simulink library "TYPEBP_MASTER_tmp"  (Simulink 8.6)
settings: Solver=ode45  StartTime=0.0  StopTime=10.0  RelTol=1e-3
undefined symbols (not defined in the file): TYPEC, TYPEC_MASTER
libraries: cdsEpicsOut x112, cdsFilt x79, cdsTP x59, cdsFiltCtrl x36, VIS_LIB x20, cdsEpicsIn x18, cdsMuxMatrix x14, STATE_BIO_MASTER x12, cdsEpicsBinIn x8, cdsFunctionCall x4, lockin x4, cdsEpicsStringIn x2
(part 1 of 13)
settings Model: Creator=controls  LastModifiedBy=controls

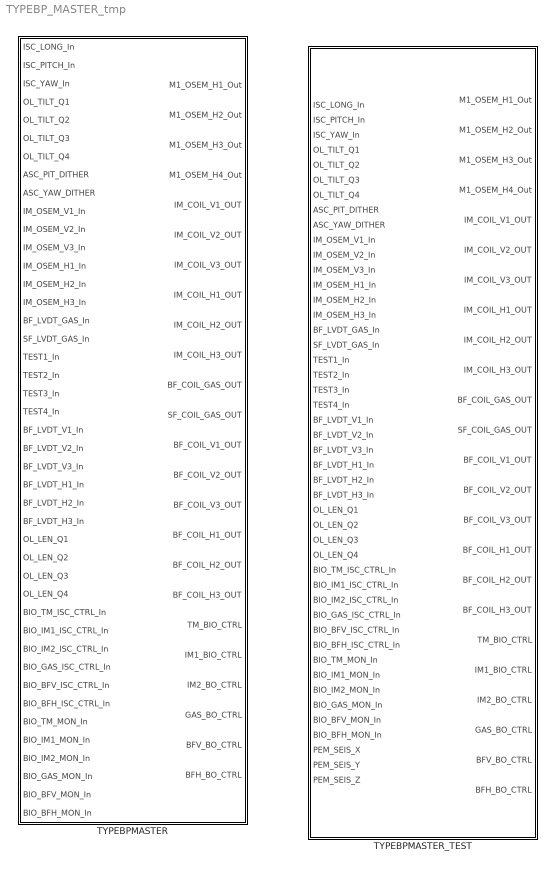
== system TYPEBP_MASTER_tmp ==
  TYPEBPMASTER : Subsystem  Description=TYPEBP MASTER  AncestorBlock=TYPEC_MASTER/TYPEC
      settings: AttributesFormatString=%<Description>
  TYPEBPMASTER_TEST : Subsystem  Description=TYPEBP MASTER
      settings: AttributesFormatString=%<Description>

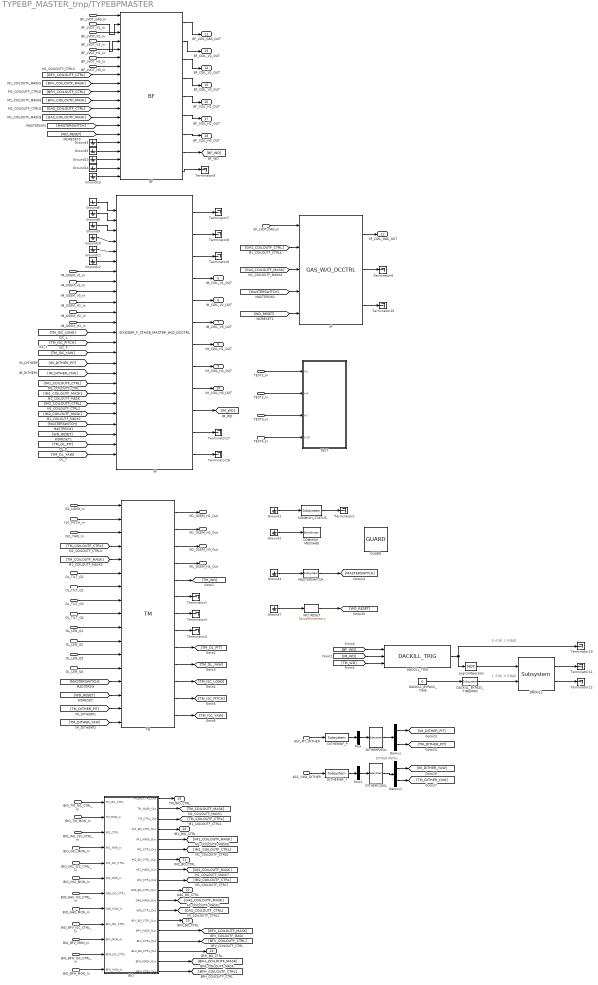
== system TYPEBP_MASTER_tmp/TYPEBPMASTER ==
  note: DITHER PATHs
      |
      |
      |
      |
      |
      |
      |
      |
      |
      |
      |
      |
      |
      |
      | .                                                                                                      .
  note: 0 if OK, 1 if BAD
  note: 1 if OK, 0 if BAD
  ISC_LONG_In : Inport
  ISC_PITCH_In : Inport  Port=2
  ISC_YAW_In : Inport  Port=3
  OL_TILT_Q1 : Inport  Port=4
  OL_TILT_Q2 : Inport  Port=5
  OL_TILT_Q3 : Inport  Port=6
  OL_TILT_Q4 : Inport  Port=7
  ASC_PIT_DITHER : Inport  Port=8
  ASC_YAW_DITHER : Inport  Port=9
  IM_OSEM_V1_In : Inport  Port=10
  IM_OSEM_V2_In : Inport  Port=11
  IM_OSEM_V3_In : Inport  Port=12
  IM_OSEM_H1_In : Inport  Port=13
  IM_OSEM_H2_In : Inport  Port=14
  IM_OSEM_H3_In : Inport  Port=15
  BF_LVDT_GAS_In : Inport  Port=16
  SF_LVDT_GAS_In : Inport  Port=17
  TEST1_In : Inport  Port=18
  TEST2_In : Inport  Port=19
  TEST3_In : Inport  Port=20
  TEST4_In : Inport  Port=21
  BF_LVDT_V1_In : Inport  Port=22
  BF_LVDT_V2_In : Inport  Port=23
  BF_LVDT_V3_In : Inport  Port=24
  BF_LVDT_H1_In : Inport  Port=25
  BF_LVDT_H2_In : Inport  Port=26
  BF_LVDT_H3_In : Inport  Port=27
  OL_LEN_Q1 : Inport  Port=28
  OL_LEN_Q2 : Inport  Port=29
  OL_LEN_Q3 : Inport  Port=30
  OL_LEN_Q4 : Inport  Port=31
  BIO_TM_ISC_CTRL_In : Inport  Port=32
  BIO_IM1_ISC_CTRL_In : Inport  Port=33
  BIO_IM2_ISC_CTRL_In : Inport  Port=34
  BIO_GAS_ISC_CTRL_In : Inport  Port=35
  BIO_BFV_ISC_CTRL_In : Inport  Port=36
  BIO_BFH_ISC_CTRL_In : Inport  Port=37
  BIO_TM_MON_In : Inport  Port=38
  BIO_IM1_MON_In : Inport  Port=39
  BIO_IM2_MON_In : Inport  Port=40
  BIO_GAS_MON_In : Inport  Port=41
  BIO_BFV_MON_In : Inport  Port=42
  BIO_BFH_MON_In : Inport  Port=43
  BF : BF_MASTER/BF
  BIO : Subsystem
  COMMISH_MESSAGE : cdsEpicsStringIn/EpicsStringIn  Tag=cdsEpicsStringIn  Description=cdsEpicsStringIn
      settings: AttributesFormatString=%<Tag>
  COMMISH_STATUS : cdsEpicsBinIn/Subsystem  Tag=cdsEpicsBinIn  Description=|
      | Purpose:                                                                            
      | Create an EPICS binary (0 or 1) input channel to the FE realtime controls.          
      |                                                                                     
      | Operation:                                                                          
      | Outputs value from an EPICS ai record. Value is binary input (bi Epics record type).
      |                                                                                     
      | Usage:                                                                              
      | Name the part with the desired EPICS channel name.
      settings: AttributesFormatString=%<Tag>
  DACKILL : cdsDacKill/Subsystem  Description=cdsDacKill
      settings: AttributesFormatString=%<Description>
  DACKILL_BYPASS_TIME : Constant  Value=0
  DACKILL_BYPASS_TIMEMON : cdsEpicsOut/Subsystem  Tag=cdsEpicsOutput  Description=|
      | Purpose:                                          
      | Output a FE signal to an EPICS channel.           
      |                                                   
      | Operation:                                        
      | Takes input value and passes it to EPICS record.  
      |                                                   
      | Usage:                                            
      | Name the part with the desired EPICS rrecord name.
      settings: AttributesFormatString=%<Tag>
  DACKILL_TRIG : VIS_LIB/DACKILL_TRIG
  DITHERINF_P : cdsFilt/Subsystem  Tag=cdsFilt  Description=|
      | Purpose:                                                                                                                                                                                                                                  
      | Standard CDS IIR filter module.                                                                                                                                                                                                           
      |                                                                                                                                                                                                                                           
      | Operation:                                                                                                                                                                                                                                
      | Consists of 10 second order section IIR filters, plus a ramped gain stage. In FE code, also provides pre-defined test points and excitation channel inputs. The filter coefficients are defined in the LIGO system using the 'foton' tool.
      |                                                                                                                                                                                                                                           
      | Usage:                                                                                                                                                                                                                                    
      | Name the part with the desired filter module name.
      settings: AttributesFormatString=%<Tag>
  DITHERINF_Y : cdsFilt/Subsystem  Tag=cdsFilt  Description=|
      | Purpose:                                                                                                                                                                                                                                  
      | Standard CDS IIR filter module.                                                                                                                                                                                                           
      |                                                                                                                                                                                                                                           
      | Operation:                                                                                                                                                                                                                                
      | Consists of 10 second order section IIR filters, plus a ramped gain stage. In FE code, also provides pre-defined test points and excitation channel inputs. The filter coefficients are defined in the LIGO system using the 'foton' tool.
      |                                                                                                                                                                                                                                           
      | Usage:                                                                                                                                                                                                                                    
      | Name the part with the desired filter module name.
      settings: AttributesFormatString=%<Tag>
  DITHERP2EUL : cdsMuxMatrix/Subsystem  Tag=cdsMuxMatrix  Description=Any size matrix. Inputs and outputs must be connected using Mux and Demux parts.
      settings: AttributesFormatString=%<Tag>
  DITHERY2EUL : cdsMuxMatrix/Subsystem  Tag=cdsMuxMatrix  Description=Any size matrix. Inputs and outputs must be connected using Mux and Demux parts.
      settings: AttributesFormatString=%<Tag>
  Demux : Demux  Outputs=2
  Demux1 : Demux  Outputs=2
  GUARD : ISC_common/GUARD
  Ground{1..15} (15 alike) : Ground
  IM : SIXOSEM_F_STAGE_MASTER/SIXOSEM_F_STAGE_MASTER_W//O_DCCTRL  Description=SIXOSEMSTAGE_FACE_MASTER
  LogicalOperator : Logic  Operator=NOT  AllPortsSameDT=off  OutDataTypeStr=boolean
  MASTERSWITCH : cdsEpicsBinIn/Subsystem  Tag=cdsEpicsBinIn  Description=|
      | Purpose:                                                                            
      | Create an EPICS binary (0 or 1) input channel to the FE realtime controls.          
      |                                                                                     
      | Operation:                                                                          
      | Outputs value from an EPICS ai record. Value is binary input (bi Epics record type).
      |                                                                                     
      | Usage:                                                                              
      | Name the part with the desired EPICS channel name.
      settings: AttributesFormatString=%<Tag>
  Mux : Mux  Inputs=1
  Mux1 : Mux  Inputs=1
  SF : GAS_MASTER/GAS_W//O_DCCTRL
  TEST : Subsystem
  TM : TM_MASTER/TM
  Terminator{1..12,17..19} (15 alike) : Terminator
  WD_RESET : cdsEpicsMomentary/EpicsMomentary  Tag=cdsEpicsMomentary
      settings: AttributesFormatString=%<Tag>
  M1_OSEM_H1_Out : Outport
  M1_OSEM_H2_Out : Outport  Port=2
  M1_OSEM_H3_Out : Outport  Port=3
  M1_OSEM_H4_Out : Outport  Port=4
  IM_COIL_V1_OUT : Outport  Port=5
  IM_COIL_V2_OUT : Outport  Port=6
  IM_COIL_V3_OUT : Outport  Port=7
  IM_COIL_H1_OUT : Outport  Port=8
  IM_COIL_H2_OUT : Outport  Port=9
  IM_COIL_H3_OUT : Outport  Port=10
  BF_COIL_GAS_OUT : Outport  Port=11
  SF_COIL_GAS_OUT : Outport  Port=12
  BF_COIL_V1_OUT : Outport  Port=13
  BF_COIL_V2_OUT : Outport  Port=14
  BF_COIL_V3_OUT : Outport  Port=15
  BF_COIL_H1_OUT : Outport  Port=16
  BF_COIL_H2_OUT : Outport  Port=17
  BF_COIL_H3_OUT : Outport  Port=18
  TM_BIO_CTRL : Outport  Port=19
  IM1_BIO_CTRL : Outport  Port=20
  IM2_BO_CTRL : Outport  Port=21
  GAS_BO_CTRL : Outport  Port=22
  BFV_BO_CTRL : Outport  Port=23
  BFH_BO_CTRL : Outport  Port=24
  wires:
  [TM_COILOUTF_MASK] -> TM/5
  [TM_COILOUTF_CTRL] -> TM/4
  [WD_RESET] -> TM/15
  WD_RESET/1 -> [WD_RESET]
  Ground7/1 -> WD_RESET/1
  TM/6 -> Terminator1/1
  TM/7 -> Terminator3/1
  TM/8 -> Terminator4/1
  [MASTERSWITCH] -> TM/14
  OL_TILT_Q4/1 -> TM/9
  ISC_YAW_In/1 -> TM/3
  ISC_PITCH_In/1 -> TM/2
  OL_TILT_Q3/1 -> TM/8
  OL_TILT_Q2/1 -> TM/7
  OL_TILT_Q1/1 -> TM/6
  Ground4/1 -> MASTERSWITCH/1
  MASTERSWITCH/1 -> [MASTERSWITCH]
  TM/4 -> M1_OSEM_H4_Out/1
  TM/3 -> M1_OSEM_H3_Out/1
  TM/2 -> M1_OSEM_H2_Out/1
  TM/5 -> [TM_WD]
  ISC_LONG_In/1 -> TM/1
  Ground2/1 -> COMMISH_MESSAGE/1
  COMMISH_STATUS/1 -> Terminator2/1
  Ground1/1 -> COMMISH_STATUS/1
  ASC_YAW_DITHER/1 -> DITHERINF_Y/1
  Mux/1 -> DITHERP2EUL/1
  DITHERP2EUL/1 -> Demux/1
  ASC_PIT_DITHER/1 -> DITHERINF_P/1
  Mux1/1 -> DITHERY2EUL/1
  DITHERY2EUL/1 -> Demux1/1
  Demux/1 -> [IM_DITHER_PIT]
  Demux/2 -> [TM_DITHER_PIT]
  Demux1/1 -> [IM_DITHER_YAW]
  Demux1/2 -> [TM_DITHER_YAW]
  DITHERINF_P/1 -> Mux/1
  DITHERINF_Y/1 -> Mux1/1
  [TM_DITHER_PIT] -> TM/16
  [TM_DITHER_YAW] -> TM/17
  Ground9/1 -> IM/3
  Ground11/1 -> IM/5
  Ground6/1 -> IM/1
  Ground8/1 -> IM/2
  [TM_ISC_LONG] -> IM/13
  Ground10/1 -> IM/4
  Ground12/1 -> IM/6
  [TM_ISC_PITCH] -> IM/14
  [TM_ISC_YAW] -> IM/15
  IM/1 -> Terminator7/1
  IM/10 -> [IM_WD]
  IM/11 -> Terminator17/1
  IM/2 -> Terminator8/1
  IM/3 -> Terminator9/1
  IM/12 -> Terminator18/1
  IM_OSEM_V3_In/1 -> IM/9
  IM_OSEM_V2_In/1 -> IM/8
  IM_OSEM_V1_In/1 -> IM/7
  IM_OSEM_H3_In/1 -> IM/12
  IM_OSEM_H2_In/1 -> IM/11
  IM_OSEM_H1_In/1 -> IM/10
  IM/4 -> IM_COIL_V1_OUT/1
  IM/5 -> IM_COIL_V2_OUT/1
  IM/6 -> IM_COIL_V3_OUT/1
  IM/7 -> IM_COIL_H1_OUT/1
  IM/8 -> IM_COIL_H2_OUT/1
  IM/9 -> IM_COIL_H3_OUT/1
  TEST3_In/1 -> TEST/3(In7)
  TEST2_In/1 -> TEST/2(In4)
  TEST1_In/1 -> TEST/1(In1)
  TEST4_In/1 -> TEST/4(In10)
  TM/1 -> M1_OSEM_H1_Out/1
  [TM_WD] -> DACKILL_TRIG/3
  DACKILL_TRIG/1 -> Terminator19/1, LogicalOperator/1
  LogicalOperator/1 -> DACKILL/1
  DACKILL_BYPASS_TIMEMON/1 -> DACKILL/2
  DACKILL_BYPASS_TIME/1 -> DACKILL_BYPASS_TIMEMON/1
  DACKILL/1 -> Terminator11/1
  DACKILL/2 -> Terminator12/1
  [IM_WD] -> DACKILL_TRIG/2
  [IM1_COILOUTF_CTRL] -> IM/18
  [IM_DITHER_PIT] -> IM/16
  [IM_DITHER_YAW] -> IM/17
  [IM1_COILOUTF_MASK] -> IM/19
  TM/9 -> [TM_OL_PIT]
  TM/10 -> [TM_OL_YAW]
  [BF_WD] -> DACKILL_TRIG/1
  OL_LEN_Q4/1 -> TM/13
  OL_LEN_Q3/1 -> TM/12
  OL_LEN_Q2/1 -> TM/11
  OL_LEN_Q1/1 -> TM/10
  [BFV_COILOUTF_MASK] -> BF/9
  [BFV_COILOUTF_CTRL] -> BF/8
  BF_LVDT_H3_In/1 -> BF/7
  BF_LVDT_H2_In/1 -> BF/6
  BF_LVDT_H1_In/1 -> BF/5
  BF_LVDT_V3_In/1 -> BF/4
  BF_LVDT_V2_In/1 -> BF/3
  BF_LVDT_V1_In/1 -> BF/2
  BF_LVDT_GAS_In/1 -> BF/1
  BF/1 -> BF_COIL_GAS_OUT/1
  BF/2 -> BF_COIL_V1_OUT/1
  BF/3 -> BF_COIL_V2_OUT/1
  BF/4 -> BF_COIL_V3_OUT/1
  BF/5 -> BF_COIL_H1_OUT/1
  BF/6 -> BF_COIL_H2_OUT/1
  BF/7 -> BF_COIL_H3_OUT/1
  BF/9 -> Terminator5/1
  BF/8 -> [BF_WD]
  [GAS_COILOUTF_CTRL] -> SF/2
  [GAS_COILOUTF_MASK] -> SF/3
  [MASTERSWITCH] -> SF/4
  [WD_RESET] -> SF/5
  SF_LVDT_GAS_In/1 -> SF/1
  SF/2 -> Terminator6/1
  SF/1 -> SF_COIL_GAS_OUT/1
  SF/3 -> Terminator10/1
  BIO/12(GAS_CTRL_Out) -> [GAS_COILOUTF_CTRL]
  BIO/11(GAS_MASK_Out) -> [GAS_COILOUTF_MASK]
  BIO/3(TM_CTRL_Out) -> [TM_COILOUTF_CTRL]
  BIO/2(TM_MASK_Out) -> [TM_COILOUTF_MASK]
  BIO/6(IM1_CTRL_Out) -> [IM1_COILOUTF_CTRL]
  BIO/5(IM1_MASK_Out) -> [IM1_COILOUTF_MASK]
  BIO/13(BFV_BO_CTRL_Out) -> BFV_BO_CTRL/1
  BIO/10(GAS_BO_CTRL_Out) -> GAS_BO_CTRL/1
  BIO/7(IM2_BO_CTRL_Out) -> IM2_BO_CTRL/1
  BIO/4(IM1_BO_CTRL_Out) -> IM1_BIO_CTRL/1
  BIO/1(TM_BO_CTRL_Out) -> TM_BIO_CTRL/1
  BIO_GAS_MON_In/1 -> BIO/8(GAS_MON_In)
  BIO_GAS_ISC_CTRL_In/1 -> BIO/7(GAS_ISC_CTRL)
  BIO_IM2_MON_In/1 -> BIO/6(IM2_MON_In)
  BIO_IM2_ISC_CTRL_In/1 -> BIO/5(IM2_ISC_CTRL)
  BIO_IM1_MON_In/1 -> BIO/4(IM1_MON_In)
  BIO_IM1_ISC_CTRL_In/1 -> BIO/3(IM1_CTRL)
  BIO_TM_MON_In/1 -> BIO/2(TM_MON_In)
  BIO_TM_ISC_CTRL_In/1 -> BIO/1(TM_ISC_CTRL)
  BIO/8(IM2_MASK_Out) -> [IM2_COILOUTF_MASK]
  BIO/9(IM2_CTRL_Out) -> [IM2_COILOUTF_CTRL]
  BIO_BFV_ISC_CTRL_In/1 -> BIO/9(BFV_ISC_CTRL)
  BIO_BFV_MON_In/1 -> BIO/10(BFV_MON_In)
  BIO_BFH_ISC_CTRL_In/1 -> BIO/11(BFH_ISC_CTRL)
  BIO_BFH_MON_In/1 -> BIO/12(BFH_MON_In)
  BIO/14(BFV_MASK_Out) -> [BFV_COILOUTF_MASK]
  BIO/15(BFV_CTRL_Out) -> [BFV_COILOUTF_CTRL]
  BIO/17(BFH_MASK_Out) -> [BFH_COILOUTF_MASK]
  BIO/18(BFH_CTRL_Out) -> [BFH_COILOUTF_CTRL]
  BIO/16(BFH_BO_CTRL_Out) -> BFH_BO_CTRL/1
  [MASTERSWITCH] -> IM/22
  [WD_RESET] -> IM/23
  [TM_OL_PIT] -> IM/24
  [TM_OL_YAW] -> IM/25
  [IM2_COILOUTF_CTRL] -> IM/20
  [IM2_COILOUTF_MASK] -> IM/21
  [MASTERSWITCH] -> BF/14
  [WD_RESET] -> BF/15
  [GAS_COILOUTF_MASK] -> BF/13
  [GAS_COILOUTF_CTRL] -> BF/12
  [BFH_COILOUTF_MASK] -> BF/11
  [BFH_COILOUTF_CTRL] -> BF/10
  Ground3/1 -> BF/16
  Ground5/1 -> BF/17
  Ground13/1 -> BF/18
  TM/11 -> [TM_ISC_LONG]
  TM/12 -> [TM_ISC_PITCH]
  TM/13 -> [TM_ISC_YAW]
  Ground14/1 -> BF/19
  Ground15/1 -> BF/20

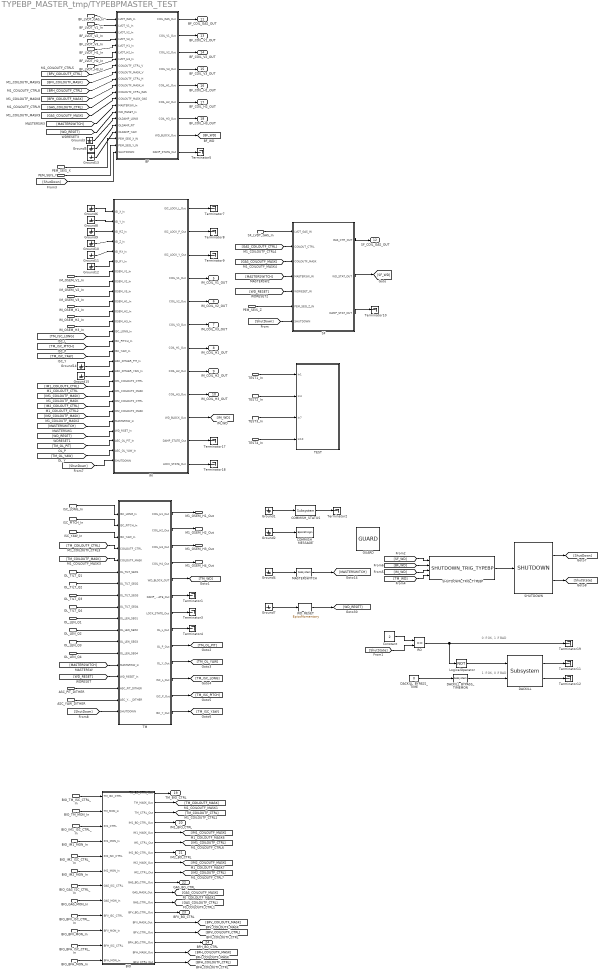
== system TYPEBP_MASTER_tmp/TYPEBPMASTER_TEST ==
  note: 1 if OK, 0 if BAD
  note: 0 if OK, 1 if BAD
  ISC_LONG_In : Inport
  ISC_PITCH_In : Inport  Port=2
  ISC_YAW_In : Inport  Port=3
  OL_TILT_Q1 : Inport  Port=4
  OL_TILT_Q2 : Inport  Port=5
  OL_TILT_Q3 : Inport  Port=6
  OL_TILT_Q4 : Inport  Port=7
  ASC_PIT_DITHER : Inport  Port=8
  ASC_YAW_DITHER : Inport  Port=9
  IM_OSEM_V1_In : Inport  Port=10
  IM_OSEM_V2_In : Inport  Port=11
  IM_OSEM_V3_In : Inport  Port=12
  IM_OSEM_H1_In : Inport  Port=13
  IM_OSEM_H2_In : Inport  Port=14
  IM_OSEM_H3_In : Inport  Port=15
  BF_LVDT_GAS_In : Inport  Port=16
  SF_LVDT_GAS_In : Inport  Port=17
  TEST1_In : Inport  Port=18
  TEST2_In : Inport  Port=19
  TEST3_In : Inport  Port=20
  TEST4_In : Inport  Port=21
  BF_LVDT_V1_In : Inport  Port=22
  BF_LVDT_V2_In : Inport  Port=23
  BF_LVDT_V3_In : Inport  Port=24
  BF_LVDT_H1_In : Inport  Port=25
  BF_LVDT_H2_In : Inport  Port=26
  BF_LVDT_H3_In : Inport  Port=27
  OL_LEN_Q1 : Inport  Port=28
  OL_LEN_Q2 : Inport  Port=29
  OL_LEN_Q3 : Inport  Port=30
  OL_LEN_Q4 : Inport  Port=31
  BIO_TM_ISC_CTRL_In : Inport  Port=32
  BIO_IM1_ISC_CTRL_In : Inport  Port=33
  BIO_IM2_ISC_CTRL_In : Inport  Port=34
  BIO_GAS_ISC_CTRL_In : Inport  Port=35
  BIO_BFV_ISC_CTRL_In : Inport  Port=36
  BIO_BFH_ISC_CTRL_In : Inport  Port=37
  BIO_TM_MON_In : Inport  Port=38
  BIO_IM1_MON_In : Inport  Port=39
  BIO_IM2_MON_In : Inport  Port=40
  BIO_GAS_MON_In : Inport  Port=41
  BIO_BFV_MON_In : Inport  Port=42
  BIO_BFH_MON_In : Inport  Port=43
  PEM_SEIS_X : Inport  Port=44
  PEM_SEIS_Y : Inport  Port=45
  PEM_SEIS_Z : Inport  Port=46
  BF : Subsystem  AncestorBlock=BF_MASTER/BF
  BIO : Subsystem
  COMMISH_MESSAGE : cdsEpicsStringIn/EpicsStringIn  Tag=cdsEpicsStringIn  Description=cdsEpicsStringIn
      settings: AttributesFormatString=%<Tag>
  COMMISH_STATUS : cdsEpicsBinIn/Subsystem  Tag=cdsEpicsBinIn  Description=|
      | Purpose:                                                                            
      | Create an EPICS binary (0 or 1) input channel to the FE realtime controls.          
      |                                                                                     
      | Operation:                                                                          
      | Outputs value from an EPICS ai record. Value is binary input (bi Epics record type).
      |                                                                                     
      | Usage:                                                                              
      | Name the part with the desired EPICS channel name.
      settings: AttributesFormatString=%<Tag>
  Constant : Constant  Value=2
  DACKILL : cdsDacKill/Subsystem  Description=cdsDacKill
      settings: AttributesFormatString=%<Description>
  DACKILL_BYPASS_TIME : Constant  Value=0
  DACKILL_BYPASS_TIMEMON : cdsEpicsOut/Subsystem  Tag=cdsEpicsOutput  Description=|
      | Purpose:                                          
      | Output a FE signal to an EPICS channel.           
      |                                                   
      | Operation:                                        
      | Takes input value and passes it to EPICS record.  
      |                                                   
      | Usage:                                            
      | Name the part with the desired EPICS rrecord name.
      settings: AttributesFormatString=%<Tag>
  GUARD : ISC_common/GUARD
  Ground{1..15} (15 alike) : Ground
  IM : Subsystem  Description=SIXOSEMSTAGE_FACE_MASTER  AncestorBlock=SIXOSEM_F_STAGE_MASTER/SIXOSEM_F_STAGE_MASTER_WO_DCCTRL
  LogicalOperator : Logic  Operator=NOT  AllPortsSameDT=off  OutDataTypeStr=boolean
  MASTERSWITCH : cdsEpicsBinIn/Subsystem  Tag=cdsEpicsBinIn  Description=|
      | Purpose:                                                                            
      | Create an EPICS binary (0 or 1) input channel to the FE realtime controls.          
      |                                                                                     
      | Operation:                                                                          
      | Outputs value from an EPICS ai record. Value is binary input (bi Epics record type).
      |                                                                                     
      | Usage:                                                                              
      | Name the part with the desired EPICS channel name.
      settings: AttributesFormatString=%<Tag>
  RO : RelationalOperator  Operator===  OutDataTypeStr=boolean
  SF : Subsystem
  SHUTDOWN : SHUTDOWN/SHUTDOWN
  SHUTDOWN_TRIG_TYPEBP : VIS_LIB/SHUTDOWN_TRIG_TYPEBP
  TEST : Subsystem
  TM : Subsystem  AncestorBlock=TM_MASTER/TM
  Terminator{1..5,7..12,17..19} (14 alike) : Terminator
  WD_RESET : cdsEpicsMomentary/EpicsMomentary  Tag=cdsEpicsMomentary
      settings: AttributesFormatString=%<Tag>
  M1_OSEM_H1_Out : Outport
  M1_OSEM_H2_Out : Outport  Port=2
  M1_OSEM_H3_Out : Outport  Port=3
  M1_OSEM_H4_Out : Outport  Port=4
  IM_COIL_V1_OUT : Outport  Port=5
  IM_COIL_V2_OUT : Outport  Port=6
  IM_COIL_V3_OUT : Outport  Port=7
  IM_COIL_H1_OUT : Outport  Port=8
  IM_COIL_H2_OUT : Outport  Port=9
  IM_COIL_H3_OUT : Outport  Port=10
  BF_COIL_GAS_OUT : Outport  Port=11
  SF_COIL_GAS_OUT : Outport  Port=12
  BF_COIL_V1_OUT : Outport  Port=13
  BF_COIL_V2_OUT : Outport  Port=14
  BF_COIL_V3_OUT : Outport  Port=15
  BF_COIL_H1_OUT : Outport  Port=16
  BF_COIL_H2_OUT : Outport  Port=17
  BF_COIL_H3_OUT : Outport  Port=18
  TM_BIO_CTRL : Outport  Port=19
  IM1_BIO_CTRL : Outport  Port=20
  IM2_BO_CTRL : Outport  Port=21
  GAS_BO_CTRL : Outport  Port=22
  BFV_BO_CTRL : Outport  Port=23
  BFH_BO_CTRL : Outport  Port=24
  wires:
  TM/13(ISC_Y_Out) -> [TM_ISC_YAW]
  TM/12(ISC_P_Out) -> [TM_ISC_PITCH]
  TM/11(ISC_L_Out) -> [TM_ISC_LONG]
  Ground13/1 -> BF/18(OLDAMP_YAW)
  Ground5/1 -> BF/17(OLDAMP_PIT)
  Ground3/1 -> BF/16(OLDAMP_LONG)
  [BFH_COILOUTF_CTRL] -> BF/10(COILOUTF_CTRL_H)
  [BFH_COILOUTF_MASK] -> BF/11(COILOUTF_MASK_H)
  [GAS_COILOUTF_CTRL] -> BF/12(COILOUTF_CTRL_GAS)
  [GAS_COILOUTF_MASK] -> BF/13(COILOUTF_MASK_GAS)
  [WD_RESET] -> BF/15(WD_RESET_In)
  [MASTERSWITCH] -> BF/14(MASTERSW_In)
  [IM2_COILOUTF_MASK] -> IM/21(IM2_COILOUTF_MASK)
  [IM2_COILOUTF_CTRL] -> IM/20(IM2_COILOUTF_CTRL)
  [TM_OL_YAW] -> IM/25(ASC_OL_YAW_In)
  [TM_OL_PIT] -> IM/24(ASC_OL_PIT_In)
  [WD_RESET] -> IM/23(WD_RSET_In)
  [MASTERSWITCH] -> IM/22(MASTERSW_In)
  BIO/16(BFH_BO_CTRL_Out) -> BFH_BO_CTRL/1
  BIO/18(BFH_CTRL_Out) -> [BFH_COILOUTF_CTRL]
  BIO/17(BFH_MASK_Out) -> [BFH_COILOUTF_MASK]
  BIO/15(BFV_CTRL_Out) -> [BFV_COILOUTF_CTRL]
  BIO/14(BFV_MASK_Out) -> [BFV_COILOUTF_MASK]
  BIO_BFH_MON_In/1 -> BIO/12(BFH_MON_In)
  BIO_BFH_ISC_CTRL_In/1 -> BIO/11(BFH_ISC_CTRL)
  BIO_BFV_MON_In/1 -> BIO/10(BFV_MON_In)
  BIO_BFV_ISC_CTRL_In/1 -> BIO/9(BFV_ISC_CTRL)
  BIO/9(IM2_CTRL_Out) -> [IM2_COILOUTF_CTRL]
  BIO/8(IM2_MASK_Out) -> [IM2_COILOUTF_MASK]
  BIO_TM_ISC_CTRL_In/1 -> BIO/1(TM_ISC_CTRL)
  BIO_TM_MON_In/1 -> BIO/2(TM_MON_In)
  BIO_IM1_ISC_CTRL_In/1 -> BIO/3(IM1_CTRL)
  BIO_IM1_MON_In/1 -> BIO/4(IM1_MON_In)
  BIO_IM2_ISC_CTRL_In/1 -> BIO/5(IM2_ISC_CTRL)
  BIO_IM2_MON_In/1 -> BIO/6(IM2_MON_In)
  BIO_GAS_ISC_CTRL_In/1 -> BIO/7(GAS_ISC_CTRL)
  BIO_GAS_MON_In/1 -> BIO/8(GAS_MON_In)
  BIO/1(TM_BO_CTRL_Out) -> TM_BIO_CTRL/1
  BIO/4(IM1_BO_CTRL_Out) -> IM1_BIO_CTRL/1
  BIO/7(IM2_BO_CTRL_Out) -> IM2_BO_CTRL/1
  BIO/10(GAS_BO_CTRL_Out) -> GAS_BO_CTRL/1
  BIO/13(BFV_BO_CTRL_Out) -> BFV_BO_CTRL/1
  BIO/5(IM1_MASK_Out) -> [IM1_COILOUTF_MASK]
  BIO/6(IM1_CTRL_Out) -> [IM1_COILOUTF_CTRL]
  BIO/2(TM_MASK_Out) -> [TM_COILOUTF_MASK]
  BIO/3(TM_CTRL_Out) -> [TM_COILOUTF_CTRL]
  BIO/11(GAS_MASK_Out) -> [GAS_COILOUTF_MASK]
  BIO/12(GAS_CTRL_Out) -> [GAS_COILOUTF_CTRL]
  SF/3(DAMP_STAT_OUT) -> Terminator10/1
  SF/1(GAS_CTR_OUT) -> SF_COIL_GAS_OUT/1
  SF/2(WD_STAT_OUT) -> [SF_WD]
  SF_LVDT_GAS_In/1 -> SF/1(LVDT_GAS_IN)
  [WD_RESET] -> SF/5(WDRESET_IN)
  [MASTERSWITCH] -> SF/4(MASTERSW_IN)
  [GAS_COILOUTF_MASK] -> SF/3(COILOUTF_MASK)
  [GAS_COILOUTF_CTRL] -> SF/2(COILOUT_CTRL)
  BF/8(WD_BLOCK_Out) -> [BF_WD]
  BF/9(DAMP_STATE_Out) -> Terminator5/1
  BF/7(COIL_H3_Out) -> BF_COIL_H3_OUT/1
  BF/6(COIL_H2_Out) -> BF_COIL_H2_OUT/1
  BF/5(COIL_H1_Out) -> BF_COIL_H1_OUT/1
  BF/4(COIL_V3_Out) -> BF_COIL_V3_OUT/1
  BF/3(COIL_V2_Out) -> BF_COIL_V2_OUT/1
  BF/2(COIL_V1_Out) -> BF_COIL_V1_OUT/1
  BF/1(COIL_GAS_Out) -> BF_COIL_GAS_OUT/1
  BF_LVDT_GAS_In/1 -> BF/1(LVDT_GAS_In)
  BF_LVDT_V1_In/1 -> BF/2(LVDT_V1_In)
  BF_LVDT_V2_In/1 -> BF/3(LVDT_V2_In)
  BF_LVDT_V3_In/1 -> BF/4(LVDT_V3_In)
  BF_LVDT_H1_In/1 -> BF/5(LVDT_H1_In)
  BF_LVDT_H2_In/1 -> BF/6(LVDT_H2_In)
  BF_LVDT_H3_In/1 -> BF/7(LVDT_H3_In)
  [BFV_COILOUTF_CTRL] -> BF/8(COILOUTF_CTRL_V)
  [BFV_COILOUTF_MASK] -> BF/9(COILOUTF_MASK_V)
  OL_LEN_Q1/1 -> TM/10(OL_LEN_SEG1)
  OL_LEN_Q2/1 -> TM/11(OL_LEN_SEG2)
  OL_LEN_Q3/1 -> TM/12(OL_LEN_SEG3)
  OL_LEN_Q4/1 -> TM/13(OL_LEN_SEG4)
  TM/10(OL_Y_Out) -> [TM_OL_YAW]
  TM/9(OL_P_Out) -> [TM_OL_PIT]
  [IM1_COILOUTF_MASK] -> IM/19(IM1_COILOUTF_MASK)
  Ground15/1 -> IM/17(ASC_DITHER_YAW_In)
  Ground14/1 -> IM/16(ASC_DITHER_PIT_In)
  [IM1_COILOUTF_CTRL] -> IM/18(IM1_COILOUTF_CTRL)
  DACKILL/2 -> Terminator12/1
  DACKILL/1 -> Terminator11/1
  DACKILL_BYPASS_TIME/1 -> DACKILL_BYPASS_TIMEMON/1
  DACKILL_BYPASS_TIMEMON/1 -> DACKILL/2
  LogicalOperator/1 -> DACKILL/1
  RO/1 -> LogicalOperator/1, Terminator19/1
  TM/1(COIL_H1_Out) -> M1_OSEM_H1_Out/1
  TEST4_In/1 -> TEST/4(In10)
  TEST1_In/1 -> TEST/1(In1)
  TEST2_In/1 -> TEST/2(In4)
  TEST3_In/1 -> TEST/3(In7)
  IM/9(COIL_H3_Out) -> IM_COIL_H3_OUT/1
  IM/8(COIL_H2_Out) -> IM_COIL_H2_OUT/1
  IM/7(COIL_H1_Out) -> IM_COIL_H1_OUT/1
  IM/6(COIL_V3_Out) -> IM_COIL_V3_OUT/1
  IM/5(COIL_V2_Out) -> IM_COIL_V2_OUT/1
  IM/4(COIL_V1_Out) -> IM_COIL_V1_OUT/1
  IM_OSEM_H1_In/1 -> IM/10(OSEM_H1_In)
  IM_OSEM_H2_In/1 -> IM/11(OSEM_H2_In)
  IM_OSEM_H3_In/1 -> IM/12(OSEM_H3_In)
  IM_OSEM_V1_In/1 -> IM/7(OSEM_V1_In)
  IM_OSEM_V2_In/1 -> IM/8(OSEM_V2_In)
  IM_OSEM_V3_In/1 -> IM/9(OSEM_V3_In)
  IM/12(LOCK_STATE_Out) -> Terminator18/1
  IM/3(ISC_LOCK_Y_Out) -> Terminator9/1
  IM/2(ISC_LOCK_P_Out) -> Terminator8/1
  IM/11(DAMP_STATE_Out) -> Terminator17/1
  IM/10(WD_BLOCK_Out) -> [IM_WD]
  IM/1(ISC_LOCK_L_Out) -> Terminator7/1
  [TM_ISC_YAW] -> IM/15(ISC_YAW_In)
  [TM_ISC_PITCH] -> IM/14(ISC_PITCH_In)
  Ground12/1 -> IM/6(ISI_RY_In)
  Ground10/1 -> IM/4(ISI_Z_In)
  [TM_ISC_LONG] -> IM/13(ISC_LONG_In)
  Ground8/1 -> IM/2(ISI_Y_In)
  Ground6/1 -> IM/1(ISI_X_In)
  Ground11/1 -> IM/5(ISI_RX_In)
  Ground9/1 -> IM/3(ISI_RZ_In)
  ASC_YAW_DITHER/1 -> TM/17(ASC_YAW_DITHER)
  ASC_PIT_DITHER/1 -> TM/16(ASC_PIT_DITHER)
  Ground1/1 -> COMMISH_STATUS/1
  COMMISH_STATUS/1 -> Terminator2/1
  Ground2/1 -> COMMISH_MESSAGE/1
  ISC_LONG_In/1 -> TM/1(ISC_LONG_In)
  TM/5(WD_BLOCK_OUT) -> [TM_WD]
  TM/2(COIL_H2_Out) -> M1_OSEM_H2_Out/1
  TM/3(COIL_H3_Out) -> M1_OSEM_H3_Out/1
  TM/4(COIL_H4_Out) -> M1_OSEM_H4_Out/1
  MASTERSWITCH/1 -> [MASTERSWITCH]
  Ground4/1 -> MASTERSWITCH/1
  OL_TILT_Q1/1 -> TM/6(OL_TILT_SEG1)
  OL_TILT_Q2/1 -> TM/7(OL_TILT_SEG2)
  OL_TILT_Q3/1 -> TM/8(OL_TILT_SEG3)
  ISC_PITCH_In/1 -> TM/2(ISC_PITCH_In)
  ISC_YAW_In/1 -> TM/3(ISC_YAW_In)
  OL_TILT_Q4/1 -> TM/9(OL_TILT_SEG4)
  [MASTERSWITCH] -> TM/14(MASTERSW_In)
  TM/8(OL_L_Out) -> Terminator4/1
  TM/7(LOCK_STATE_Out) -> Terminator3/1
  TM/6(DAMP_STATE_Out) -> Terminator1/1
  Ground7/1 -> WD_RESET/1
  WD_RESET/1 -> [WD_RESET]
  [WD_RESET] -> TM/15(WD_RESET_In)
  [TM_COILOUTF_CTRL] -> TM/4(COILOUTF_CTRL)
  [TM_COILOUTF_MASK] -> TM/5(COILOUTF_MASK)
  PEM_SEIS_Z/1 -> SF/6(PEM_SEIS_Z_IN)
  PEM_SEIS_X/1 -> BF/19(PEM_SEIS_X_IN)
  PEM_SEIS_Y/1 -> BF/20(PEM_SEIS_Y_IN)
  [BF_WD] -> SHUTDOWN_TRIG_TYPEBP/2
  [TM_WD] -> SHUTDOWN_TRIG_TYPEBP/4
  [IM_WD] -> SHUTDOWN_TRIG_TYPEBP/3
  SHUTDOWN_TRIG_TYPEBP/1 -> SHUTDOWN/1
  SHUTDOWN/1 -> [ShutDown]
  SHUTDOWN/2 -> [ShutState]
  Constant/1 -> RO/1
  [ShutState] -> RO/2
  [ShutDown] -> SF/7(SHUTDOWN)
  [SF_WD] -> SHUTDOWN_TRIG_TYPEBP/1
  [ShutDown] -> BF/21(SHUTDOWN)
  [ShutDown] -> IM/26(SHUTDOWN)
  [ShutDown] -> TM/18(SHUTDOWN)

== system TYPEBP_MASTER_tmp/TYPEBPMASTER/BIO ==
  note: 12 Bit Word
  note: 12 Bit Word
  note: 12 Bit Word
  note: 12 Bit Word
  note: 12 Bit Word
  TM_ISC_CTRL : Inport
  TM_MON_In : Inport  Port=2
  IM1_CTRL : Inport  Port=3
  IM1_MON_In : Inport  Port=4
  IM2_ISC_CTRL : Inport  Port=5
  IM2_MON_In : Inport  Port=6
  GAS_ISC_CTRL : Inport  Port=7
  GAS_MON_In : Inport  Port=8
  BFV_ISC_CTRL : Inport  Port=9
  BFV_MON_In : Inport  Port=10
  BFH_ISC_CTRL : Inport  Port=11
  BFH_MON_In : Inport  Port=12
  BFH : STATE_BIO_MASTER/UIM_BIO_MASTER
  BFV : STATE_BIO_MASTER/UIM_BIO_MASTER
  GAS : STATE_BIO_MASTER/UIM_BIO_MASTER
  IM1 : STATE_BIO_MASTER/UIM_BIO_MASTER
  IM2 : STATE_BIO_MASTER/UIM_BIO_MASTER
  TM : STATE_BIO_MASTER/UIM_BIO_MASTER
  TM_BO_CTRL_Out : Outport
  TM_MASK_Out : Outport  Port=2
  TM_CTRL_Out : Outport  Port=3
  IM1_BO_CTRL_Out : Outport  Port=4
  IM1_MASK_Out : Outport  Port=5
  IM1_CTRL_Out : Outport  Port=6
  IM2_BO_CTRL_Out : Outport  Port=7
  IM2_MASK_Out : Outport  Port=8
  IM2_CTRL_Out : Outport  Port=9
  GAS_BO_CTRL_Out : Outport  Port=10
  GAS_MASK_Out : Outport  Port=11
  GAS_CTRL_Out : Outport  Port=12
  BFV_BO_CTRL_Out : Outport  Port=13
  BFV_MASK_Out : Outport  Port=14
  BFV_CTRL_Out : Outport  Port=15
  BFH_BO_CTRL_Out : Outport  Port=16
  BFH_MASK_Out : Outport  Port=17
  BFH_CTRL_Out : Outport  Port=18
  wires:
  BFV/3 -> BFV_BO_CTRL_Out/1
  BFV/2 -> BFV_CTRL_Out/1
  BFV/1 -> BFV_MASK_Out/1
  GAS/3 -> GAS_BO_CTRL_Out/1
  GAS/2 -> GAS_CTRL_Out/1
  GAS/1 -> GAS_MASK_Out/1
  IM2/3 -> IM2_BO_CTRL_Out/1
  IM2/2 -> IM2_CTRL_Out/1
  IM2/1 -> IM2_MASK_Out/1
  IM1/3 -> IM1_BO_CTRL_Out/1
  IM1/2 -> IM1_CTRL_Out/1
  IM1/1 -> IM1_MASK_Out/1
  TM/3 -> TM_BO_CTRL_Out/1
  TM/2 -> TM_CTRL_Out/1
  TM/1 -> TM_MASK_Out/1
  BFV_ISC_CTRL/1 -> BFV/1
  BFV_MON_In/1 -> BFV/2
  GAS_ISC_CTRL/1 -> GAS/1
  GAS_MON_In/1 -> GAS/2
  IM2_ISC_CTRL/1 -> IM2/1
  IM2_MON_In/1 -> IM2/2
  IM1_MON_In/1 -> IM1/2
  IM1_CTRL/1 -> IM1/1
  TM_ISC_CTRL/1 -> TM/1
  TM_MON_In/1 -> TM/2
  BFH/3 -> BFH_BO_CTRL_Out/1
  BFH/2 -> BFH_CTRL_Out/1
  BFH/1 -> BFH_MASK_Out/1
  BFH_ISC_CTRL/1 -> BFH/1
  BFH_MON_In/1 -> BFH/2
